simulink model "DAQP_simulink_test"  (Simulink 9.1)
settings: Solver=FixedStepDiscrete  StartTime=0.0  StopTime=0  FixedStep=1  RelTol=1e-3
values from neighbouring files (symbols this model uses):
  A = M(ms+1:end,:)*T    [generate_test_QP.m]
  blower = dlower-M*v    [generate_test_QP.m]
  bupper = dupper-M*v    [generate_test_QP.m]
  f = T'*v    [generate_test_QP.m]
  H = T'*T    [generate_test_QP.m]
  sense = zeros(m,1,'int32')    [generate_test_QP.m]
settings Model: Creator=Chr_S  LastModifiedBy=Chr_S
settings DataIOCC: SaveFormat=Dataset  ReturnWorkspaceOutputs=on
settings OptimizationCC: LifeSpan=auto
settings DebuggingCC: UnderspecifiedInitializationDetection=Simplified  MergeDetectMultiDrivingBlocksExec=error  SFUnexpectedBacktrackingDiag=error  SFNoUnconditionalDefaultTransitionDiag=error  SFExecutionAtInitializationDiag=warning
settings HardwareCC: ProdBitPerPointer=64  ProdBitPerSizeT=64  ProdBitPerPtrDiffT=64  ProdLargestAtomicFloat=Float  ProdIntDivRoundTo=Zero  ProdEndianess=LittleEndian  ProdWordSize=64  ProdHWDeviceType=Intel->x86-64 (Windows64)
settings ModelReferenceCC: PropagateSignalLabelsOutOfModel=on
settings SFSimCC: SimUseLocalCustomCode=on
settings RTWCC: RTWUseLocalCustomCode=on
settings GRTTargetCC: TargetLangStandard=C99 (ISO)  CombineOutputUpdateFcns=on  GRTInterface=off
settings ConfigComp: CovMetricSettings=dwe  CovHtmlReporting=off  CovSaveCumulativeToWorkspaceVar=off  CovSaveSingleToWorkspaceVar=off  CovExternalEMLEnable=on

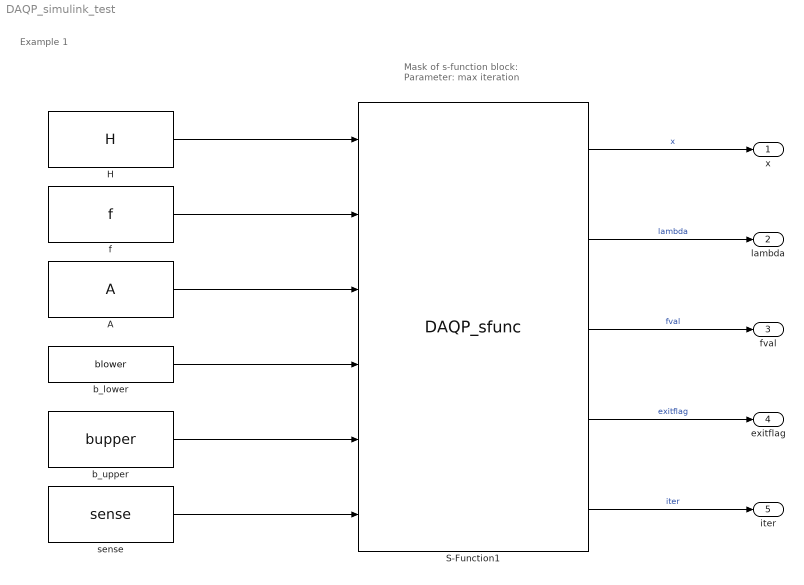
== system DAQP_simulink_test ==
  note: Example 1
  note: Mask of s-function block:
      | Parameter: max iteration
  A : Constant  Value=A  VectorParams1D=off  SampleTime=-1
  H : Constant  Value=H
  S-Function1 : S-Function  FunctionName=DAQP_sfunc  Parameters=10000,0  SFunctionDeploymentMode=off  EnableBusSupport=off
  b_lower : Constant  Value=blower
  b_upper : Constant  Value=bupper
  f : Constant  Value=f
  sense : Constant  Value=sense  OutDataTypeStr=double  SampleTime=1
  x : Outport
  lambda : Outport  Port=2
  fval : Outport  Port=3
  exitflag : Outport  Port=4
  iter : Outport  Port=5
  wires:
  S-Function1/1 -> x/1  "x"
  S-Function1/2 -> lambda/1  "lambda"
  A/1 -> S-Function1/3
  b_lower/1 -> S-Function1/4
  b_upper/1 -> S-Function1/5
  H/1 -> S-Function1/1
  f/1 -> S-Function1/2
  S-Function1/3 -> fval/1  "fval"
  S-Function1/4 -> exitflag/1  "exitflag"
  S-Function1/5 -> iter/1  "iter"
  sense/1 -> S-Function1/6
